simulink model "simulink1"  (R2020a)
settings: Solver=VariableStepAuto  StartTime=0.0  StopTime=10.0  RelTol=1e-3
settings Model: Creator=16002  LastModifiedBy=16002

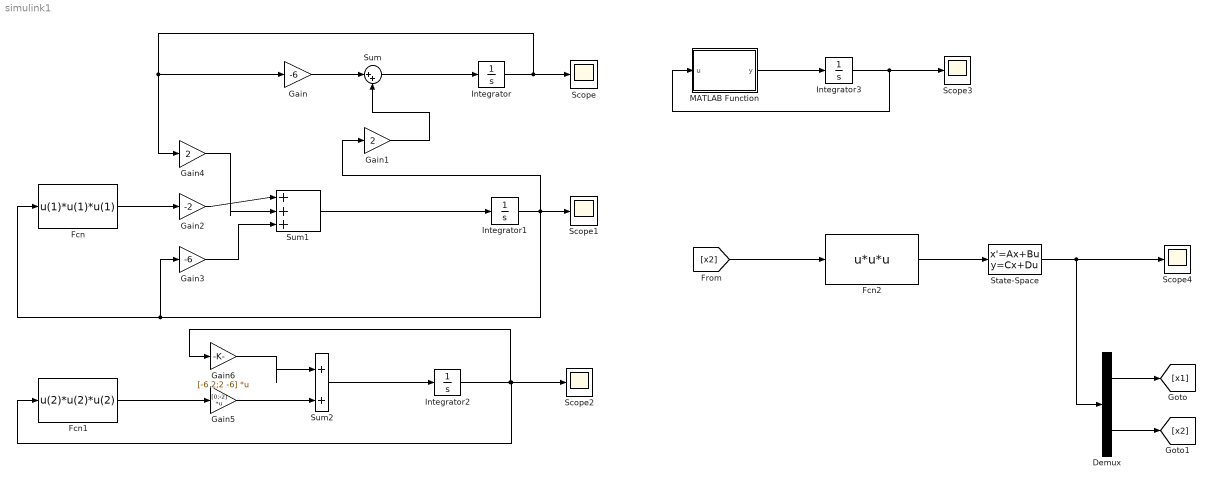
== system simulink1 ==
  Demux : Demux  Outputs=2
  Fcn : Fcn  Expr=u(1)*u(1)*u(1)
  Fcn1 : Fcn  Expr=u(2)*u(2)*u(2)
  Fcn2 : Fcn  Expr=u*u*u
  Gain : Gain  Gain=-6
  Gain1 : Gain  Gain=2
  Gain2 : Gain  Gain=-2
  Gain3 : Gain  Gain=-6
  Gain4 : Gain  Gain=2
  Gain5 : Gain  Gain=[0;-2]  Multiplication=Matrix(K*u)
  Gain6 : Gain  Gain=[-6 2;2 -6]  Multiplication=Matrix(K*u)
  Integrator : Integrator  InitialCondition=0.3
  Integrator1 : Integrator  InitialCondition=-0.1
  Integrator2 : Integrator  InitialCondition=[0.3 -0.1]
  Integrator3 : Integrator  InitialCondition=[0.3 -0.1]
  MATLAB Function : MATLAB Function  TreatAsAtomicUnit=on
  Scope{,1..4} (5 alike) : Scope
  State-Space : StateSpace  A=[-6 2;2 -6]  B=[0;-2]  C=[1 0;0 1]  D=[0;0]  InitialCondition=[0.3 -0.1]
  Sum : Sum  Inputs=|++
  Sum1 : Sum  Inputs=|+++
  Sum2 : Sum  Inputs=|++
  wires:
  Fcn/1 -> Gain2/1
  Gain4/1 -> Sum1/2
  Gain2/1 -> Sum1/1
  Gain3/1 -> Sum1/3
  Sum1/1 -> Integrator1/1
  Integrator1/1 -> Gain3/1, Fcn/1, Scope1/1, Gain1/1
  Gain/1 -> Sum/1
  Gain1/1 -> Sum/2
  Sum/1 -> Integrator/1
  Integrator/1 -> Gain4/1, Gain/1, Scope/1
  Fcn1/1 -> Gain5/1
  Gain5/1 -> Sum2/2
  Gain6/1 -> Sum2/1
  Sum2/1 -> Integrator2/1
  Integrator2/1 -> Fcn1/1, Scope2/1, Gain6/1
  Integrator3/1 -> MATLAB Function/1(u), Scope3/1
  MATLAB Function/1(y) -> Integrator3/1
  State-Space/1 -> Demux/1, Scope4/1
  Fcn2/1 -> State-Space/1
  [x2] -> Fcn2/1
  Demux/1 -> [x1]
  Demux/2 -> [x2]

== matlab function simulink1/MATLAB Function ==
  data: u input; y output
function y = fcn(u)
% x1=u(1);
% x2=u(2);
% dx1=-6*x1+2*x2;
% dx2=2*x1-6*x2-2*x2^3;
% y=[dx1,dx2];
y=[-6 2;2 -6]*u+[0;-2]*u(2)^3
